simulink model "sample"  (R2016b)
settings: Solver=VariableStepAuto  StartTime=0.0  StopTime=10.0  RelTol=1e-3
libraries: dsparch4 x1
settings Model: Creator=zhangjin  LastModifiedBy=zhangjin

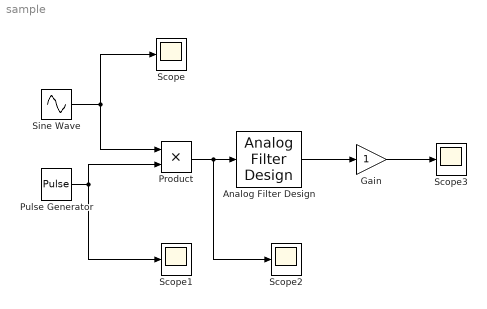
== system sample ==
  Analog Filter Design : dsparch4/Analog Filter Design  method=Butterworth  filttype=Lowpass  N=8  Wlo=30  Whi=80  Rp=2  Rs=40
  Gain : Gain
  Product : Product
  Pulse Generator : DiscretePulseGenerator  PulseType=Time based  Period=10  PulseWidth=5
  Scope{,1..3} (4 alike) : Scope
  Sine Wave : Sin  SampleTime=0
  wires:
  Sine Wave/1 -> Scope/1, Product/1
  Pulse Generator/1 -> Scope1/1, Product/2
  Product/1 -> Scope2/1, Analog Filter Design/1
  Analog Filter Design/1 -> Gain/1
  Gain/1 -> Scope3/1
